simulink model "practise1"  (R2017b)
settings: Solver=VariableStepAuto  StartTime=0.0  StopTime=10.0  RelTol=1e-3
values from neighbouring files (symbols this model uses):
  a0 = 0.02005    [mode.m]
  a2 = -0.00505    [mode.m]
  g = 9.81    [mode.m]
  I = m1*r1^2+m2*r2^2+m3*r3^2    (= 0.0258852375)    [mode.m]
  m1 = 0.233    [mode.m]
  m2 = 0.145    [mode.m]
  m3 = 0.125    [mode.m]
  p0 = 0    [mode.m]
  p1 = 0.2851    [mode.m]
  p2 = -0.0105    [mode.m]
  r1 = 0.2475    [mode.m]
  r2 = 0.2175    [mode.m]
  r3 = 0.1950    (= 0.195)    [mode.m]
settings Model: Creator=Usuario  LastModifiedBy=Usuario

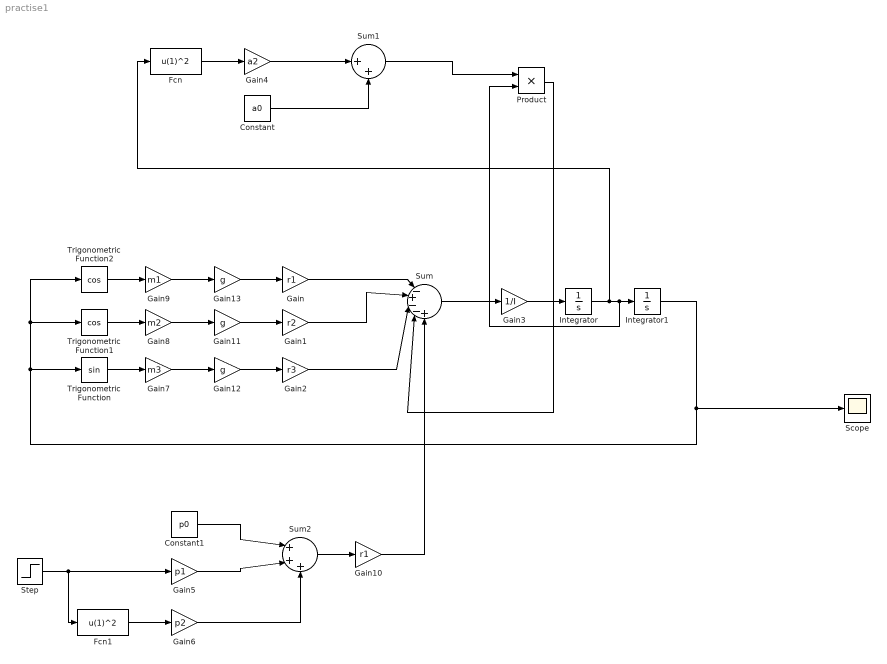
== system practise1 ==
  Constant : Constant  Value=a0
  Constant1 : Constant  Value=p0
  Fcn : Fcn  Expr=u(1)^2
  Fcn1 : Fcn  Expr=u(1)^2
  Gain : Gain  Gain=r1
  Gain1 : Gain  Gain=r2
  Gain10 : Gain  Gain=r1
  Gain11 : Gain  Gain=g
  Gain12 : Gain  Gain=g
  Gain13 : Gain  Gain=g
  Gain2 : Gain  Gain=r3
  Gain3 : Gain  Gain=1/I
  Gain4 : Gain  Gain=a2
  Gain5 : Gain  Gain=p1
  Gain6 : Gain  Gain=p2
  Gain7 : Gain  Gain=m3
  Gain8 : Gain  Gain=m2
  Gain9 : Gain  Gain=m1
  Integrator : Integrator
  Integrator1 : Integrator
  Product : Product
  Scope : Scope
  Step : Step  Before=4  After=10  SampleTime=0
  Sum : Sum  Inputs=|-+--+
  Sum1 : Sum  Inputs=|++
  Sum2 : Sum  Inputs=|+++
  Trigonometric Function : Trigonometry
  Trigonometric Function1 : Trigonometry  Operator=cos
  Trigonometric Function2 : Trigonometry  Operator=cos
  wires:
  Trigonometric Function1/1 -> Gain8/1
  Trigonometric Function2/1 -> Gain9/1
  Trigonometric Function/1 -> Gain7/1
  Gain8/1 -> Gain11/1
  Gain2/1 -> Sum/3
  Gain1/1 -> Sum/2
  Gain/1 -> Sum/1
  Integrator1/1 -> Scope/1, Trigonometric Function2/1, Trigonometric Function1/1, Trigonometric Function/1
  Gain3/1 -> Integrator/1
  Sum/1 -> Gain3/1
  Gain4/1 -> Sum1/1
  Constant/1 -> Sum1/2
  Fcn/1 -> Gain4/1
  Integrator/1 -> Fcn/1, Product/2, Integrator1/1
  Sum1/1 -> Product/1
  Product/1 -> Sum/4
  Step/1 -> Fcn1/1, Gain5/1
  Fcn1/1 -> Gain6/1
  Constant1/1 -> Sum2/1
  Gain5/1 -> Sum2/2
  Gain6/1 -> Sum2/3
  Sum2/1 -> Gain10/1
  Gain10/1 -> Sum/5
  Gain11/1 -> Gain1/1
  Gain7/1 -> Gain12/1
  Gain12/1 -> Gain2/1
  Gain9/1 -> Gain13/1
  Gain13/1 -> Gain/1
